simulink model "ACC_speed_change_curve_cs"  (R2016a)
settings: Solver=ode5  SolverMode=SingleTasking  StartTime=0.0  StopTime=inf  FixedStep=1/1000  RelTol=1e-3
PreLoadFcn:
  | mbxruntime.callbacks.PreLoadFcn(bdroot);
  | check_NUTS_defined;
  | 
  | assignin('base',['model_closed_' bdroot],false);addpath('../includes_ACC');
PostLoadFcn:
  | mbxruntime.callbacks.PostLoadFcn(bdroot);
InitFcn:
  | mbxruntime.callbacks.InitFcn(bdroot);
StartFcn:
  | mbxruntime.callbacks.StartFcn(bdroot);
StopFcn:
  | mbxruntime.callbacks.StopFcn(bdroot);
model workspace (MAT data in the model file):
  mbox_table : struct (value not decoded)
  model_closed = 0
  sim_status = 0
undefined symbols (not defined in the file or in its folder): DiscIntNeverNeededParam
undefined symbols (not defined in the file): SteeringColumn, SteeringWheel, WheelL0, WheelL1, WheelR0, WheelR1
libraries: simulink_extras x49, simulink x29, PreScanSimulinkLibrary x24, PreScanUsefulBlocks x2, Solver_SF x1, simulink_need_slupdate x1
(part 16 of 17)

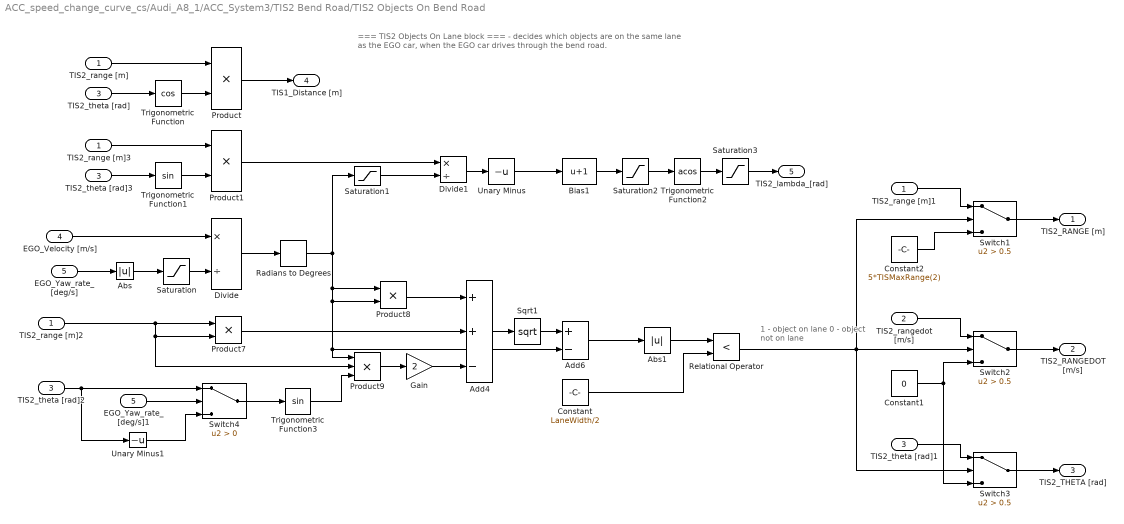
== system ACC_speed_change_curve_cs/Audi_A8_1/ACC_System3/TIS2 Bend Road/TIS2 Objects On Bend Road ==
  note: === TIS2 Objects On Lane block ===
      |
      |  - decides which objects are on the same lane as the EGO car,
      |     when the EGO car drives through the bend road.
  note: 1  - object      on lane
      | 0 - object not on lane
  TIS2_range [m] : Inport
  TIS2_rangedot [m/s] : Inport  Port=2
  TIS2_theta [rad] : Inport  Port=3
  EGO_Velocity [m/s] : Inport  Port=4
  EGO_Yaw_rate_[deg/s] : Inport  Port=5
  Abs : Abs
  Abs1 : Abs
  Add4 : Sum  Inputs=++-
  Add6 : Sum  Inputs=+-
  Bias1 : Bias  Bias=1
  Constant : Constant  Value=LaneWidth/2
  Constant1 : Constant  Value=0
  Constant2 : Constant  Value=5*TISMaxRange(2)
  Divide : Product  Inputs=*/
  Divide1 : Product  Inputs=*/
  EGO_Yaw_rate_[deg/s]1 : InportShadow  Port=5
  Gain : Gain  Gain=2
  Product{,1,7..8} (4 alike) : Product  RndMeth=Zero
  Product9 : Product  Inputs=3  RndMeth=Zero
  Radians to Degrees : simulink_extras/Transformations/Radians to Degrees
  Relational Operator : RelationalOperator  Operator=<  OutDataTypeStr=boolean
  Saturation : Saturate  UpperLimit=inf  LowerLimit=1e-6
  Saturation1 : Saturate  UpperLimit=inf  LowerLimit=1e-6
  Saturation2 : Saturate  UpperLimit=1  LowerLimit=-1
  Saturation3 : Saturate  UpperLimit=pi  LowerLimit=0
  Sqrt1 : Math  Operator=sqrt  SaturateOnIntegerOverflow=on
  Switch1 : Switch  Criteria=u2 > Threshold  Threshold=0.5
  Switch2 : Switch  Criteria=u2 > Threshold  Threshold=0.5
  Switch3 : Switch  Criteria=u2 > Threshold  Threshold=0.5
  Switch4 : Switch  Criteria=u2 > Threshold
  TIS2_range [m]1 : InportShadow
  TIS2_range [m]2 : InportShadow
  TIS2_range [m]3 : InportShadow
  TIS2_theta [rad]1 : InportShadow  Port=3
  TIS2_theta [rad]2 : InportShadow  Port=3
  TIS2_theta [rad]3 : InportShadow  Port=3
  Trigonometric Function : Trigonometry  Operator=cos
  Trigonometric Function1 : Trigonometry
  Trigonometric Function2 : Trigonometry  Operator=acos
  Trigonometric Function3 : Trigonometry
  Unary Minus : UnaryMinus
  Unary Minus1 : UnaryMinus
  TIS2_RANGE [m] : Outport
  TIS2_RANGEDOT [m/s] : Outport  Port=2
  TIS2_THETA [rad] : Outport  Port=3
  TIS1_Distance [m] : Outport  Port=4
  TIS2_lambda_[rad] : Outport  Port=5
  wires:
  Abs/1 -> Saturation/1
  Saturation3/1 -> TIS2_lambda_[rad]/1
  Saturation2/1 -> Trigonometric Function2/1
  Saturation1/1 -> Divide1/2
  Saturation/1 -> Divide/2
  Constant/1 -> Relational Operator/2
  Abs1/1 -> Relational Operator/1
  Product1/1 -> Divide1/1
  TIS2_theta [rad]3/1 -> Trigonometric Function1/1
  TIS2_range [m]3/1 -> Product1/1
  TIS2_range [m]2/1 -> Product9/2, Product7/2, Product7/1
  Unary Minus1/1 -> Switch4/3
  TIS2_theta [rad]2/1 -> Unary Minus1/1, Switch4/1
  Switch4/1 -> Trigonometric Function3/1
  EGO_Yaw_rate_[deg/s]1/1 -> Switch4/2
  Add6/1 -> Abs1/1
  Sqrt1/1 -> Add6/1
  Add4/1 -> Sqrt1/1
  Trigonometric Function3/1 -> Product9/3
  Product9/1 -> Gain/1
  Gain/1 -> Add4/3
  Product7/1 -> Add4/2
  Product8/1 -> Add4/1
  Product/1 -> TIS1_Distance [m]/1
  Trigonometric Function2/1 -> Saturation3/1
  Unary Minus/1 -> Bias1/1
  Divide1/1 -> Unary Minus/1
  Bias1/1 -> Saturation2/1
  Switch3/1 -> TIS2_THETA [rad]/1
  Switch2/1 -> TIS2_RANGEDOT [m/s]/1
  Switch1/1 -> TIS2_RANGE [m]/1
  Constant2/1 -> Switch1/3
  Constant1/1 -> Switch3/3, Switch2/3
  TIS2_theta [rad]1/1 -> Switch3/1
  TIS2_range [m]1/1 -> Switch1/1
  TIS2_rangedot [m/s]/1 -> Switch2/1
  Relational Operator/1 -> Switch3/2, Switch2/2, Switch1/2
  Radians to Degrees/1 -> Saturation1/1, Add6/2, Product9/1, Product8/2, Product8/1
  Divide/1 -> Radians to Degrees/1
  EGO_Yaw_rate_[deg/s]/1 -> Abs/1
  EGO_Velocity [m/s]/1 -> Divide/1
  Trigonometric Function1/1 -> Product1/2
  Trigonometric Function/1 -> Product/2
  TIS2_theta [rad]/1 -> Trigonometric Function/1
  TIS2_range [m]/1 -> Product/1

== system ACC_speed_change_curve_cs/Audi_A8_1/ACC_System3/TIS2 Bend Road/TIS2 Sorting Fun ==
  note: === TIS1 Sorting Fun block ===
      |
      |  - transforms information from the first sensor
      |    to the more appropriate form.
  TIS2range [m] : Inport
  TIS2rangedot [m/s] : Inport  Port=2
  TIS2theta [deg] : Inport  Port=3
  Degrees to Radians : simulink_extras/Transformations/Degrees to Radians
  Switch : Switch  Criteria=u2 ~= 0
  Unary Minus : UnaryMinus
  Unary Minus1 : UnaryMinus
  range max : Constant  Value=5*TISMaxRange(2)
  TIS2_RANGE [m] : Outport
  TIS2_RANGEDOT [m/s] : Outport  Port=2
  TIS2_THETA [rad] : Outport  Port=3
  wires:
  Unary Minus1/1 -> TIS2_RANGEDOT [m/s]/1
  TIS2theta [deg]/1 -> Unary Minus/1
  TIS2range [m]/1 -> Switch/1, Switch/2
  Degrees to Radians/1 -> TIS2_THETA [rad]/1
  range max/1 -> Switch/3
  TIS2rangedot [m/s]/1 -> Unary Minus1/1
  Switch/1 -> TIS2_RANGE [m]/1
  Unary Minus/1 -> Degrees to Radians/1

== system ACC_speed_change_curve_cs/Audi_A8_1/ACC_System3/TIS2 Straight Road/Hold ==
  HWTflagIN : Inport
  lead_vel_in : Inport  Port=2
  HWTflagIN1 : InportShadow
  If : If  IfExpression=u1 < 0.1  SampleTime=Tsensor
  If Action Subsystem : Subsystem  TreatAsAtomicUnit=on
  If Action Subsystem1 : Subsystem  TreatAsAtomicUnit=on
  Merge : Merge
  HWT_flag : Outport
  wires:
  HWTflagIN1/1 -> If Action Subsystem/1(In1)
  HWTflagIN/1 -> If Action Subsystem1/1(In1)
  Merge/1 -> HWT_flag/1
  If Action Subsystem1/1(Out1) -> Merge/2
  If Action Subsystem/1(Out1) -> Merge/1
  If/2 -> If Action Subsystem1/Action
  If/1 -> If Action Subsystem/Action
  lead_vel_in/1 -> If/1

== system ACC_speed_change_curve_cs/Audi_A8_1/ACC_System3/TIS2 Straight Road/TIS2 Closest Object ==
  note: === TIS2 Closest Object block ===
      |
      |  - passing through data about potentially the most dangerous object driving on the straight road.
  TIS2_rangedot [m/s] : Inport
  TIS2_distance [m] : Inport  Port=2
  index : Inport  Port=3
  Selector1 : Selector  InputPortWidth=TISdet(2)  IndexOptions=Index vector (port)  Indices=[1 3]  OutputSizes=1
  Selector2 : Selector  InputPortWidth=TISdet(2)  IndexOptions=Index vector (port)  Indices=[1 3]  OutputSizes=1
  rangedot [m/s] : Outport
  distance [m/s] : Outport  Port=2
  wires:
  index/1 -> Selector2/2, Selector1/2
  TIS2_rangedot [m/s]/1 -> Selector1/1
  Selector1/1 -> rangedot [m/s]/1
  TIS2_distance [m]/1 -> Selector2/1
  Selector2/1 -> distance [m/s]/1

== system ACC_speed_change_curve_cs/Audi_A8_1/ACC_System3/TIS2 Straight Road/TIS2 HWT Computing ==
  note: === TIS1 HWT Computing block===
      |
      |  - computes HeadWay Time (HWT) as it is defined in ISO norms.
  Distance [m] : Inport
  HWT demanded : Inport  Port=2
  Velocity [m/s] : Inport  Port=3
  If : If
  If Action Subsystem : Subsystem  TreatAsAtomicUnit=on
  If Action Subsystem1 : Subsystem  TreatAsAtomicUnit=on
  Merge : Merge
  HWT [s] : Outport
  wires:
  HWT demanded/1 -> If Action Subsystem1/1(HWT demanded [s])
  Distance [m]/1 -> If Action Subsystem/1(Distance [m])
  Merge/1 -> HWT [s]/1
  If Action Subsystem1/1(Out1) -> Merge/2
  If Action Subsystem/1(HWT [s]) -> Merge/1
  If/2 -> If Action Subsystem1/Action
  If/1 -> If Action Subsystem/Action
  Velocity [m/s]/1 -> If Action Subsystem/2(Velocity [m/s]), If/1

== system ACC_speed_change_curve_cs/Audi_A8_1/ACC_System3/TIS2 Straight Road/TIS2 HWT Computing2 ==
  note: === TIS1 HWT Computing block===
      |
      |  - computes HeadWay Time (HWT) as it is defined in ISO norms.
  Distance [m] : Inport
  Velocity [m/s] : Inport  Port=2
  If : If
  If Action Subsystem : Subsystem  TreatAsAtomicUnit=on
  If Action Subsystem1 : Subsystem  TreatAsAtomicUnit=on
  Merge : Merge
  HWT [s] : Outport
  wires:
  Distance [m]/1 -> If Action Subsystem/1(Distance [m])
  Merge/1 -> HWT [s]/1
  If Action Subsystem1/1(Out1) -> Merge/2
  If Action Subsystem/1(HWT [s]) -> Merge/1
  If/2 -> If Action Subsystem1/Action
  If/1 -> If Action Subsystem/Action
  Velocity [m/s]/1 -> If Action Subsystem/2(Velocity [m/s]), If/1

== system ACC_speed_change_curve_cs/Audi_A8_1/ACC_System3/TIS2 Straight Road/TIS2 HWT Flag ==
  note: === TIS2 HWT Flag block ===
      |
      |  - outputs the HeadWay Time (HWT) flag,
      |  - holds a high level if the criteria were met,
      |  - sets HWT flag to low level if leading car
      |    went outside the scope of the sensors.
  Distance closest [m] : Inport
  HWT_dem [s] : Inport  Port=2
  HWT [s] : Inport  Port=3
  Standstill distance : Inport  Port=4
  Abs : Abs
  Compare To Constant1 : simulink/Logic and Bit Operations/Compare To Constant  relop===  const=5*TISMaxRange(2)  OutDataTypeStr=uint8
  Constant : Constant
  Constant1 : Constant  Value=0
  Data Type Conversion : DataTypeConversion
  Data Type Conversion1 : DataTypeConversion
  Discrete-Time Integrator : DiscreteIntegrator  ExternalReset=level  SampleTime=Tsensor  ICPrevOutput=DiscIntNeverNeededParam  ICPrevScaledInput=DiscIntNeverNeededParam
  Distance closest [m]1 : InportShadow
  Gain : Gain  Gain=2
  Gain1 : Gain
  Gain2 : Gain  Gain=1e6  OutDataTypeStr=double
  Gain3 : Gain  Gain=1e6  OutDataTypeStr=double
  Gain4 : Gain  Gain=1.25
  Gain6 : Gain  Gain=100
  Gain7 : Gain  Gain=1.25
  Gain8 : Gain  Gain=0.01
  HWT [s]1 : InportShadow  Port=3
  HWT [s]3 : InportShadow  Port=3
  HWT_dem [s]1 : InportShadow  Port=2
  HWT_dem [s]2 : InportShadow  Port=2
  Logical Operator : Logic  AllPortsSameDT=off  OutDataTypeStr=boolean
  Logical Operator1 : Logic  AllPortsSameDT=off  OutDataTypeStr=boolean
  Logical Operator2 : Logic  Operator=OR  Inputs=3  AllPortsSameDT=off  OutDataTypeStr=boolean
  Logical Operator3 : Logic  AllPortsSameDT=off  OutDataTypeStr=boolean
  MinMax : MinMax
  MinMax2 : MinMax
  Relational Operator : RelationalOperator  Operator=<=  OutDataTypeStr=boolean
  Relational Operator1 : RelationalOperator  OutDataTypeStr=boolean
  Relational Operator2 : RelationalOperator  Operator=>  OutDataTypeStr=boolean
  Relational Operator4 : RelationalOperator  Operator=>  OutDataTypeStr=boolean
  Rounding Function : Rounding
  Sum of Elements : Sum  Inputs=+
  Switch : Switch  Criteria=u2 > Threshold
  HWT_flag : Outport
  wires:
  Data Type Conversion1/1 -> Gain3/1
  Data Type Conversion/1 -> Gain2/1
  Relational Operator4/1 -> Logical Operator2/3
  Gain7/1 -> Relational Operator4/2
  Gain8/1 -> Relational Operator4/1
  MinMax2/1 -> Gain6/1
  Rounding Function/1 -> Gain8/1
  Gain6/1 -> Rounding Function/1
  HWT [s]3/1 -> MinMax2/1
  HWT_dem [s]2/1 -> Gain7/1
  Gain4/1 -> Relational Operator/2
  Switch/1 -> HWT_flag/1
  Constant1/1 -> Switch/3
  Constant/1 -> Switch/1
  Abs/1 -> Switch/2
  Discrete-Time Integrator/1 -> Abs/1
  Gain3/1 -> Discrete-Time Integrator/1
  Gain2/1 -> Discrete-Time Integrator/2
  Logical Operator3/1 -> Logical Operator2/2
  MinMax/1 -> Logical Operator3/1
  Relational Operator2/1 -> Logical Operator3/2
  Standstill distance/1 -> Relational Operator2/2
  Distance closest [m]1/1 -> Relational Operator2/1
  HWT_dem [s]1/1 -> Gain/1
  Logical Operator2/1 -> Data Type Conversion/1
  Gain1/1 -> MinMax/1
  Relational Operator1/1 -> Gain1/1
  Gain/1 -> Relational Operator1/2
  HWT [s]1/1 -> Relational Operator1/1
  Compare To Constant1/1 -> Logical Operator1/1, Logical Operator1/2
  HWT [s]/1 -> Relational Operator/1
  HWT_dem [s]/1 -> Gain4/1
  Relational Operator/1 -> Sum of Elements/1
  Sum of Elements/1 -> Logical Operator/1, Logical Operator/2
  Logical Operator/1 -> Data Type Conversion1/1
  Distance closest [m]/1 -> Compare To Constant1/1
  Logical Operator1/1 -> Logical Operator2/1

== system ACC_speed_change_curve_cs/Audi_A8_1/ACC_System3/TIS2 Straight Road/TIS2 Lead Car Longitudinal Velocity ==
  note: === TIS2 Lead Car Longitudinal Velocity block ===
      |
      |  - computes the leading car absolute velocity and safe distance between the EGO and leading car.
  HWT_dem (s) : Inport
  TIS2 Rangedot [m/s] : Inport  Port=2
  EGO Velocity [m/s] : Inport  Port=3
  Standstill [m] : Inport  Port=4
  Abs : Abs
  Add : Sum  Inputs=+-
  Constant : Constant  Value=0
  Divide : Product  Inputs=*/
  HWT_dem (s)1 : InportShadow
  Product : Product  RndMeth=Zero
  Relational Operator : RelationalOperator  Operator=<=  OutDataTypeStr=boolean
  Switch : Switch  Criteria=u2 > Threshold
  Switch1 : Switch  Criteria=u2 ~= 0
  TIS2 Rangedot [m/s]1 : InportShadow  Port=2
  Safe distance [m] : Outport
  Lead velocity [m/s] : Outport  Port=2
  wires:
  Abs/1 -> Switch1/1, Relational Operator/1, Product/1
  TIS2 Rangedot [m/s]1/1 -> Switch1/2
  Switch1/1 -> Lead velocity [m/s]/1
  Constant/1 -> Switch1/3
  EGO Velocity [m/s]/1 -> Add/1
  TIS2 Rangedot [m/s]/1 -> Add/2
  Add/1 -> Abs/1
  HWT_dem (s)/1 -> Product/2
  Product/1 -> Switch/3
  Switch/1 -> Safe distance [m]/1
  Standstill [m]/1 -> Divide/1, Switch/1
  HWT_dem (s)1/1 -> Divide/2
  Divide/1 -> Relational Operator/2
  Relational Operator/1 -> Switch/2

== system ACC_speed_change_curve_cs/Audi_A8_1/ACC_System3/TIS2 Straight Road/TIS2 Objects On Lane ==
  note: === TIS2 Objects On Lane block ===
      |
      |  - decides which objects are on the same lane as the EGO car,
      |    when the EGO car drives straight.
  TIS2_range [m] : Inport
  TIS2_rangedot [m/s] : Inport  Port=2
  TIS2_theta [rad] : Inport  Port=3
  Abs : Abs
  Compare To Constant : simulink/Logic and Bit Operations/Compare To Constant  relop=<  const=LaneWidth/2  OutDataTypeStr=boolean
  Constant : Constant  Value=0
  Product : Product  RndMeth=Zero
  Product1 : Product  RndMeth=Zero
  Switch1 : Switch  Criteria=u2 > Threshold  Threshold=0.5
  Switch3 : Switch  Criteria=u2 > Threshold  Threshold=0.5
  TIS2 range max (higher value) : Constant  Value=5*TISMaxRange(2)
  Trigonometric Function : Trigonometry
  Trigonometric Function1 : Trigonometry  Operator=cos
  TIS2_RANGEDOT [m/s] : Outport
  TIS2_Distance [m] : Outport  Port=2
  wires:
  TIS2_theta [rad]/1 -> Abs/1, Trigonometric Function1/1
  Trigonometric Function/1 -> Product/2
  Product/1 -> Compare To Constant/1
  TIS2_range [m]/1 -> Product1/1, Product/1
  TIS2_rangedot [m/s]/1 -> Switch1/1
  Switch1/1 -> TIS2_RANGEDOT [m/s]/1
  Switch3/1 -> TIS2_Distance [m]/1
  Abs/1 -> Trigonometric Function/1
  Trigonometric Function1/1 -> Product1/2
  Product1/1 -> Switch3/1
  TIS2 range max (higher value)/1 -> Switch3/3
  Constant/1 -> Switch1/3
  Compare To Constant/1 -> Switch3/2, Switch1/2

== system ACC_speed_change_curve_cs/Audi_A8_1/ACC_System3/TIS2 Straight Road/TIS2 Sorting Fun ==
  note: === TIS2 Sorting Fun block ===
      |
      |  - transforms information from the second sensor
      |    to the more appropriate form.
  TIS2range [m] : Inport
  TIS2rangedot [m/s] : Inport  Port=2
  TIS2theta [deg] : Inport  Port=3
  Degrees to Radians : simulink_extras/Transformations/Degrees to Radians
  Switch : Switch  Criteria=u2 ~= 0
  Unary Minus : UnaryMinus
  Unary Minus1 : UnaryMinus
  range max (higher value which will not generate high level of HWT flag) : Constant  Value=5*TISMaxRange(2)
  TIS2_RANGE [m] : Outport
  TIS2_RANGEDOT [m/s] : Outport  Port=2
  TIS2_THETA [rad] : Outport  Port=3
  wires:
  Unary Minus/1 -> Degrees to Radians/1
  Switch/1 -> TIS2_RANGE [m]/1
  TIS2rangedot [m/s]/1 -> Unary Minus1/1
  range max (higher value which will not generate high level of HWT flag)/1 -> Switch/3
  Degrees to Radians/1 -> TIS2_THETA [rad]/1
  TIS2range [m]/1 -> Switch/1, Switch/2
  TIS2theta [deg]/1 -> Unary Minus/1
  Unary Minus1/1 -> TIS2_RANGEDOT [m/s]/1

== system ACC_speed_change_curve_cs/Audi_A8_1/CarSim2PreScan/Transformation_WheelGlobal2WheelLocal/Subsystem ==
  Wheels_Pos_Global_xyz_[m] : Inport
  In2 : Inport  Port=2
  In3 : Inport  Port=3
  In4 : Inport  Port=4
  Demux1 : Demux  Outputs=[3 3 3 3]
  Dot Product{1..12} (12 alike) : DotProduct  InputSameDT=on  OutDataTypeStr=Inherit: Inherit via internal rule
  Mux{1..4} (4 alike) : Mux  Inputs=3
  FL_xyz : Outport
  FR_xyz : Outport  Port=2
  RL_xyz : Outport  Port=3
  RR_xyz : Outport  Port=4
  wires:
  [ThirdRow] -> Dot Product12/2
  [ThirdRow] -> Dot Product9/2
  [ThirdRow] -> Dot Product6/2
  [SecondRow] -> Dot Product11/2
  [SecondRow] -> Dot Product8/2
  [SecondRow] -> Dot Product5/2
  In2/1 -> [FirstRow], Dot Product1/2
  [FirstRow] -> Dot Product10/2
  [FirstRow] -> Dot Product7/2
  [FirstRow] -> Dot Product4/2
  Demux1/4 -> Dot Product12/1, Dot Product10/1, Dot Product11/1
  Demux1/3 -> Dot Product9/1, Dot Product7/1, Dot Product8/1
  Demux1/2 -> Dot Product6/1, Dot Product5/1, Dot Product4/1
  Demux1/1 -> Dot Product3/1, Dot Product2/1, Dot Product1/1
  Mux4/1 -> RR_xyz/1
  Dot Product11/1 -> Mux4/2
  Dot Product12/1 -> Mux4/3
  Dot Product10/1 -> Mux4/1
  Mux3/1 -> RL_xyz/1
  Dot Product8/1 -> Mux3/2
  Dot Product9/1 -> Mux3/3
  Dot Product7/1 -> Mux3/1
  Mux1/1 -> FR_xyz/1
  Dot Product5/1 -> Mux1/2
  Dot Product6/1 -> Mux1/3
  Dot Product4/1 -> Mux1/1
  Mux2/1 -> FL_xyz/1
  Dot Product2/1 -> Mux2/2
  Dot Product3/1 -> Mux2/3
  Dot Product1/1 -> Mux2/1
  Wheels_Pos_Global_xyz_[m]/1 -> Demux1/1
  In4/1 -> [ThirdRow], Dot Product3/2
  In3/1 -> [SecondRow], Dot Product2/2

== system ACC_speed_change_curve_cs/Audi_A8_1/PathFollower_1/CTRL REFERENCES/Calculate Preview Point (pvp) by extrapolating current Vehicle Position (p0) with Preview Distance and Vehicle Orientation ==
  Preview Distance : Inport
  x,y,Y Demux [m,m,rad] : Inport  Port=2
  Demux : Demux  Outputs=3
  Fcn : Fcn  Expr=u(2)*cos(u(1))
  Fcn1 : Fcn  Expr=u(2)*sin(u(1))
  Mux : Mux  Inputs=2
  Sum : Sum  Inputs=|++
  Sum1 : Sum  Inputs=|++
  x_glob_PVD : Outport
  y_glob_PVD : Outport  Port=2
  Y [rad] : Outport  Port=3
  wires:
  Demux/3 -> Mux/1, Y [rad]/1
  Demux/1 -> Sum/1
  Demux/2 -> Sum1/1
  Preview Distance/1 -> Mux/2
  Mux/1 -> Fcn/1, Fcn1/1
  Fcn/1 -> Sum/2
  Fcn1/1 -> Sum1/2
  Sum/1 -> x_glob_PVD/1
  Sum1/1 -> y_glob_PVD/1
  x,y,Y Demux [m,m,rad]/1 -> Demux/1

== system ACC_speed_change_curve_cs/Audi_A8_1/PathFollower_1/CTRL REFERENCES/Find Reference Point (pref) on Trajectory closest to PVP Point (pvp) ==
  In1 : Inport
  In2 : Inport  Port=2
  In3 : Inport  Port=3
  In4 : Inport  Port=4
  eml_find_closest_trajectory_points : MATLAB Function  TreatAsAtomicUnit=on
  Out1 : Outport
  Out2 : Outport  Port=2
  Out3 : Outport  Port=3
  wires:
  eml_find_closest_trajectory_points/3(Actor_traj_angle) -> Out3/1
  eml_find_closest_trajectory_points/2(Actor_traj_distance) -> Out2/1
  eml_find_closest_trajectory_points/1(pref) -> Out1/1
  In1/1 -> eml_find_closest_trajectory_points/1(pvp)
  In2/1 -> eml_find_closest_trajectory_points/2(TrajOffset_x_y_Y)
  In3/1 -> eml_find_closest_trajectory_points/3(ActorOffset_Left_Right)
  In4/1 -> eml_find_closest_trajectory_points/4(p0)

== system ACC_speed_change_curve_cs/Audi_A8_1/PathFollower_1/DELTA CTRL/Calculate preview angle ==
  In1 : Inport
  In2 : Inport  Port=2
  In3 : Inport  Port=3
  eml_preview_angle_and_distance : MATLAB Function  TreatAsAtomicUnit=on
  Out1 : Outport
  wires:
  In3/1 -> eml_preview_angle_and_distance/3(p0)
  In2/1 -> eml_preview_angle_and_distance/2(pref)
  In1/1 -> eml_preview_angle_and_distance/1(pvp)
  eml_preview_angle_and_distance/1(alpha) -> Out1/1

== system ACC_speed_change_curve_cs/Audi_A8_1/PathFollower_1/DELTA CTRL/Error check ==
  Add3 : Sum  Inputs=-+
  Demux : Demux  Outputs=2
  Selector1 : Selector  InputPortWidth=3  IndexOptions=Index vector (dialog)  Indices=[1 2]  OutputSizes=1
  p0_x error : Scope
  p0_y error : Scope
  wires:
  Demux/2 -> p0_y error/1
  Add3/1 -> Demux/1
  Demux/1 -> p0_x error/1
  [pref0] -> Add3/2
  [p0] -> Selector1/1
  Selector1/1 -> Add3/1

== system ACC_speed_change_curve_cs/Audi_A8_1/PathFollower_1/THROTTLE CTRL/If Desired Velocity = 0 ==
  In1 : Inport
  Action Port : ActionPort  InitializeStates=reset  PropagateVarSize=During execution  ActionType=then
  constant : Constant  Value=0
  constant1 : Constant  Value=150
  throttle [%] : Outport  InitialOutput=[0]
  brake pressure [bar] : Outport  Port=2  InitialOutput=[150]
  Auto_GearShift : Outport  Port=3
  wires:
  constant1/1 -> brake pressure [bar]/1
  constant/1 -> throttle [%]/1
  In1/1 -> Auto_GearShift/1

== system ACC_speed_change_curve_cs/Audi_A8_1/PathFollower_1/THROTTLE CTRL/If Desired Velocity ~= 0 ==
  note: CONSTANT VELOCITY CONTROL
  note: No brake/throttle actions
      | in case of small ctrl error,
      |  in order to prevent nervous
      | ctrl behaviour
  In1 : Inport
  Desired Velocity [m/s] : Inport  Port=2
  Action Port : ActionPort  InitializeStates=reset  PropagateVarSize=During execution  ActionType=else
  Dead Zone : DeadZone  LowerValue=-10  UpperValue=1  SaturateOnIntegerOverflow=on
  Gain11 : Gain  Gain=10
  Gain6 : Gain  Gain=-1
  Limiter_brake : Saturate  UpperLimit=150  LowerLimit=0
  Limiter_throttle : Saturate  UpperLimit=100  LowerLimit=0
  PID Controller : simulink_need_slupdate/PID Controller  P=20  I=0.3  D=3.065
  throttle [%] : Outport
  brake pressure [bar] : Outport  Port=2
  Auto_GearShift : Outport  Port=3
  wires:
  Limiter_throttle/1 -> throttle [%]/1  "throttle"
  Limiter_brake/1 -> brake pressure [bar]/1
  Gain6/1 -> Limiter_brake/1
  Gain11/1 -> Gain6/1
  Dead Zone/1 -> Limiter_throttle/1, Gain11/1
  Desired Velocity [m/s]/1 -> PID Controller/1
  PID Controller/1 -> Dead Zone/1
  In1/1 -> Auto_GearShift/1

== system ACC_speed_change_curve_cs/Audi_A8_1/SELF_Demux/compas converter/cart2compas ==
  Angle [deg] : Inport
  Constant : Constant  Value=90
  Constant1 : Constant  Value=360
  Gain : Gain  Gain=1/360
  Gain1 : Gain  Gain=360
  Gain2 : Gain  Gain=-1
  Rounding Function : Rounding
  Sum : Sum  Inputs=|-+
  Sum1 : Sum  Inputs=-+|
  Sum2 : Sum  Inputs=++|
  heading [deg] : Outport
  wires:
  Gain/1 -> Rounding Function/1
  Rounding Function/1 -> Gain1/1
  Gain1/1 -> Sum/1
  Angle [deg]/1 -> Sum1/2
  Sum/1 -> Gain2/1
  Sum1/1 -> Gain/1, Sum/2
  Constant/1 -> Sum1/1
  Gain2/1 -> Sum2/2
  Constant1/1 -> Sum2/1
  Sum2/1 -> heading [deg]/1

== system ACC_speed_change_curve_cs/Audi_A8_1/Trajectories/Traj2State1/Traj2State2 ==
  traj : Inport
  MuxState : Subsystem
  Traj2MuxState_Ext : Subsystem
  state : Outport
  wires:
  Traj2MuxState_Ext/9(Y [rad]) -> MuxState/9(Y [rad])
  Traj2MuxState_Ext/8(P [rad]) -> MuxState/8(P [rad])
  Traj2MuxState_Ext/7(R [rad]) -> MuxState/7(R [rad])
  Traj2MuxState_Ext/6(dz [m/s]) -> MuxState/6(dz [m/s])
  Traj2MuxState_Ext/5(dy [m/s]) -> MuxState/5(dy [m/s])
  Traj2MuxState_Ext/4(dx [m/s]) -> MuxState/4(dx [m/s])
  Traj2MuxState_Ext/3(z [m]) -> MuxState/3(z [m])
  Traj2MuxState_Ext/2(y [m]) -> MuxState/2(y [m])
  Traj2MuxState_Ext/1(x [m]) -> MuxState/1(x [m])
  MuxState/1(state) -> state/1
  traj/1 -> Traj2MuxState_Ext/1(Traj)

== system ACC_speed_change_curve_cs/BMW_X5_1/SELF_Demux/compas converter/cart2compas ==
  Angle [deg] : Inport
  Constant : Constant  Value=90
  Constant1 : Constant  Value=360
  Gain : Gain  Gain=1/360
  Gain1 : Gain  Gain=360
  Gain2 : Gain  Gain=-1
  Rounding Function : Rounding
  Sum : Sum  Inputs=|-+
  Sum1 : Sum  Inputs=-+|
  Sum2 : Sum  Inputs=++|
  heading [deg] : Outport
  wires:
  Gain/1 -> Rounding Function/1
  Rounding Function/1 -> Gain1/1
  Gain1/1 -> Sum/1
  Angle [deg]/1 -> Sum1/2
  Sum/1 -> Gain2/1
  Sum1/1 -> Gain/1, Sum/2
  Constant/1 -> Sum1/1
  Gain2/1 -> Sum2/2
  Constant1/1 -> Sum2/1
  Sum2/1 -> heading [deg]/1

== system ACC_speed_change_curve_cs/BMW_X5_1/Trajectories/Traj2State1/Traj2State2 ==
  traj : Inport
  MuxState : Subsystem
  Traj2MuxState_Ext : Subsystem
  state : Outport
  wires:
  Traj2MuxState_Ext/9(Y [rad]) -> MuxState/9(Y [rad])
  Traj2MuxState_Ext/8(P [rad]) -> MuxState/8(P [rad])
  Traj2MuxState_Ext/7(R [rad]) -> MuxState/7(R [rad])
  Traj2MuxState_Ext/6(dz [m/s]) -> MuxState/6(dz [m/s])
  Traj2MuxState_Ext/5(dy [m/s]) -> MuxState/5(dy [m/s])
  Traj2MuxState_Ext/4(dx [m/s]) -> MuxState/4(dx [m/s])
  Traj2MuxState_Ext/3(z [m]) -> MuxState/3(z [m])
  Traj2MuxState_Ext/2(y [m]) -> MuxState/2(y [m])
  Traj2MuxState_Ext/1(x [m]) -> MuxState/1(x [m])
  MuxState/1(state) -> state/1
  traj/1 -> Traj2MuxState_Ext/1(Traj)

== system ACC_speed_change_curve_cs/Toyota_Previa_1/SELF_Demux/compas converter/cart2compas ==
  Angle [deg] : Inport
  Constant : Constant  Value=90
  Constant1 : Constant  Value=360
  Gain : Gain  Gain=1/360
  Gain1 : Gain  Gain=360
  Gain2 : Gain  Gain=-1
  Rounding Function : Rounding
  Sum : Sum  Inputs=|-+
  Sum1 : Sum  Inputs=-+|
  Sum2 : Sum  Inputs=++|
  heading [deg] : Outport
  wires:
  Gain/1 -> Rounding Function/1
  Rounding Function/1 -> Gain1/1
  Gain1/1 -> Sum/1
  Angle [deg]/1 -> Sum1/2
  Sum/1 -> Gain2/1
  Sum1/1 -> Gain/1, Sum/2
  Constant/1 -> Sum1/1
  Gain2/1 -> Sum2/2
  Constant1/1 -> Sum2/1
  Sum2/1 -> heading [deg]/1

== system ACC_speed_change_curve_cs/Toyota_Previa_1/Trajectories/Traj2State1/Traj2State2 ==
  traj : Inport
  MuxState : Subsystem
  Traj2MuxState_Ext : Subsystem
  state : Outport
  wires:
  Traj2MuxState_Ext/9(Y [rad]) -> MuxState/9(Y [rad])
  Traj2MuxState_Ext/8(P [rad]) -> MuxState/8(P [rad])
  Traj2MuxState_Ext/7(R [rad]) -> MuxState/7(R [rad])
  Traj2MuxState_Ext/6(dz [m/s]) -> MuxState/6(dz [m/s])
  Traj2MuxState_Ext/5(dy [m/s]) -> MuxState/5(dy [m/s])
  Traj2MuxState_Ext/4(dx [m/s]) -> MuxState/4(dx [m/s])
  Traj2MuxState_Ext/3(z [m]) -> MuxState/3(z [m])
  Traj2MuxState_Ext/2(y [m]) -> MuxState/2(y [m])
  Traj2MuxState_Ext/1(x [m]) -> MuxState/1(x [m])
  MuxState/1(state) -> state/1
  traj/1 -> Traj2MuxState_Ext/1(Traj)

== system ACC_speed_change_curve_cs/Toyota_Yaris_1/SELF_Demux/compas converter/cart2compas ==
  Angle [deg] : Inport
  Constant : Constant  Value=90
  Constant1 : Constant  Value=360
  Gain : Gain  Gain=1/360
  Gain1 : Gain  Gain=360
  Gain2 : Gain  Gain=-1
  Rounding Function : Rounding
  Sum : Sum  Inputs=|-+
  Sum1 : Sum  Inputs=-+|
  Sum2 : Sum  Inputs=++|
  heading [deg] : Outport
  wires:
  Gain/1 -> Rounding Function/1
  Rounding Function/1 -> Gain1/1
  Gain1/1 -> Sum/1
  Angle [deg]/1 -> Sum1/2
  Sum/1 -> Gain2/1
  Sum1/1 -> Gain/1, Sum/2
  Constant/1 -> Sum1/1
  Gain2/1 -> Sum2/2
  Constant1/1 -> Sum2/1
  Sum2/1 -> heading [deg]/1

== system ACC_speed_change_curve_cs/Toyota_Yaris_1/Trajectories/Traj2State1/Traj2State2 ==
  traj : Inport
  MuxState : Subsystem
  Traj2MuxState_Ext : Subsystem
  state : Outport
  wires:
  Traj2MuxState_Ext/9(Y [rad]) -> MuxState/9(Y [rad])
  Traj2MuxState_Ext/8(P [rad]) -> MuxState/8(P [rad])
  Traj2MuxState_Ext/7(R [rad]) -> MuxState/7(R [rad])
  Traj2MuxState_Ext/6(dz [m/s]) -> MuxState/6(dz [m/s])
  Traj2MuxState_Ext/5(dy [m/s]) -> MuxState/5(dy [m/s])
  Traj2MuxState_Ext/4(dx [m/s]) -> MuxState/4(dx [m/s])
  Traj2MuxState_Ext/3(z [m]) -> MuxState/3(z [m])
  Traj2MuxState_Ext/2(y [m]) -> MuxState/2(y [m])
  Traj2MuxState_Ext/1(x [m]) -> MuxState/1(x [m])
  MuxState/1(state) -> state/1
  traj/1 -> Traj2MuxState_Ext/1(Traj)

== system ACC_speed_change_curve_cs/Audi_A8_1/ACC_System/TIS1 Bend Road/Hold/If Action Subsystem ==
  In1 : Inport
  Action Port : ActionPort  InitializeStates=reset  PropagateVarSize=During execution  ActionType=then
  Constant : Constant
  Constant1 : Constant  Value=0
  Discrete-Time Integrator : DiscreteIntegrator  gainval=100  InitialConditionSource=external  InitialConditionSetting=State (most efficient)  SampleTime=Tsensor  LimitOutput=on  UpperSaturationLimit=1  LowerSaturationLimit=0  ICPrevOutput=DiscIntNeverNeededParam  ICPrevScaledInput=DiscIntNeverNeededParam
  Gain3 : Gain  Gain=1e6  OutDataTypeStr=double
  Switch : Switch  Criteria=u2 > Threshold
  Out1 : Outport
  wires:
  Gain3/1 -> Discrete-Time Integrator/1
  In1/1 -> Gain3/1, Switch/2
  Discrete-Time Integrator/1 -> Out1/1
  Switch/1 -> Discrete-Time Integrator/2
  Constant/1 -> Switch/1
  Constant1/1 -> Switch/3

== system ACC_speed_change_curve_cs/Audi_A8_1/ACC_System/TIS1 Bend Road/Hold/If Action Subsystem1 ==
  In1 : Inport
  Action Port : ActionPort  PropagateVarSize=During execution  ActionType=else
  Out1 : Outport
  wires:
  In1/1 -> Out1/1

== system ACC_speed_change_curve_cs/Audi_A8_1/ACC_System/TIS1 Bend Road/TIS1 HWT Computing/If Action Subsystem ==
  Distance [m] : Inport
  Velocity [m/s] : Inport  Port=2
  Action Port : ActionPort  PropagateVarSize=During execution  ActionType=then
  Product : Product  Inputs=*/  RndMeth=Zero
  HWT [s] : Outport
  wires:
  Distance [m]/1 -> Product/1
  Velocity [m/s]/1 -> Product/2
  Product/1 -> HWT [s]/1

== system ACC_speed_change_curve_cs/Audi_A8_1/ACC_System/TIS1 Bend Road/TIS1 HWT Computing/If Action Subsystem1 ==
  Action Port : ActionPort  PropagateVarSize=During execution  ActionType=else
  Constant : Constant  Value=inf
  Out1 : Outport  InitialOutput=0
  wires:
  Constant/1 -> Out1/1

== system ACC_speed_change_curve_cs/Audi_A8_1/ACC_System/TIS1 Straight Road/Hold/If Action Subsystem ==
  In1 : Inport
  Action Port : ActionPort  InitializeStates=reset  PropagateVarSize=During execution  ActionType=then
  Constant : Constant
  Constant1 : Constant  Value=0
  Discrete-Time Integrator : DiscreteIntegrator  gainval=100  InitialConditionSource=external  InitialConditionSetting=State (most efficient)  SampleTime=Tsensor  LimitOutput=on  UpperSaturationLimit=1  LowerSaturationLimit=0  ICPrevOutput=DiscIntNeverNeededParam  ICPrevScaledInput=DiscIntNeverNeededParam
  Gain3 : Gain  Gain=1e6  OutDataTypeStr=double
  Switch : Switch  Criteria=u2 > Threshold
  Out1 : Outport
  wires:
  Gain3/1 -> Discrete-Time Integrator/1
  In1/1 -> Gain3/1, Switch/2
  Discrete-Time Integrator/1 -> Out1/1
  Switch/1 -> Discrete-Time Integrator/2
  Constant/1 -> Switch/1
  Constant1/1 -> Switch/3

== system ACC_speed_change_curve_cs/Audi_A8_1/ACC_System/TIS1 Straight Road/Hold/If Action Subsystem1 ==
  In1 : Inport
  Action Port : ActionPort  PropagateVarSize=During execution  ActionType=else
  Out1 : Outport
  wires:
  In1/1 -> Out1/1

== system ACC_speed_change_curve_cs/Audi_A8_1/ACC_System/TIS1 Straight Road/TIS1 HWT Computing/If Action Subsystem ==
  Distance [m] : Inport
  Velocity [m/s] : Inport  Port=2
  Action Port : ActionPort  PropagateVarSize=During execution  ActionType=then
  Product : Product  Inputs=*/  RndMeth=Zero
  HWT [s] : Outport
  wires:
  Distance [m]/1 -> Product/1
  Velocity [m/s]/1 -> Product/2
  Product/1 -> HWT [s]/1

== system ACC_speed_change_curve_cs/Audi_A8_1/ACC_System/TIS1 Straight Road/TIS1 HWT Computing/If Action Subsystem1 ==
  HWT demanded [s] : Inport
  Action Port : ActionPort  PropagateVarSize=During execution  ActionType=else
  Gain : Gain  Gain=2*ones(TISdet(1),1)
  Out1 : Outport
  wires:
  Gain/1 -> Out1/1
  HWT demanded [s]/1 -> Gain/1

== system ACC_speed_change_curve_cs/Audi_A8_1/ACC_System/TIS1 Straight Road/TIS1 HWT Computing1/If Action Subsystem ==
  Distance [m] : Inport
  Velocity [m/s] : Inport  Port=2
  Action Port : ActionPort  PropagateVarSize=During execution  ActionType=then
  Product : Product  Inputs=*/  RndMeth=Zero
  HWT [s] : Outport
  wires:
  Distance [m]/1 -> Product/1
  Velocity [m/s]/1 -> Product/2
  Product/1 -> HWT [s]/1

== system ACC_speed_change_curve_cs/Audi_A8_1/ACC_System/TIS1 Straight Road/TIS1 HWT Computing1/If Action Subsystem1 ==
  Action Port : ActionPort  PropagateVarSize=During execution  ActionType=else
  Constant : Constant  Value=inf
  Out1 : Outport  InitialOutput=0
  wires:
  Constant/1 -> Out1/1

== system ACC_speed_change_curve_cs/Audi_A8_1/ACC_System/TIS2 Bend Road/Hold/If Action Subsystem ==
  In1 : Inport
  Action Port : ActionPort  InitializeStates=reset  PropagateVarSize=During execution  ActionType=then
  Constant : Constant
  Constant1 : Constant  Value=0
  Discrete-Time Integrator : DiscreteIntegrator  gainval=100  InitialConditionSource=external  InitialConditionSetting=State (most efficient)  SampleTime=Tsensor  LimitOutput=on  UpperSaturationLimit=1  LowerSaturationLimit=0  ICPrevOutput=DiscIntNeverNeededParam  ICPrevScaledInput=DiscIntNeverNeededParam
  Gain3 : Gain  Gain=1e6  OutDataTypeStr=double
  Switch : Switch  Criteria=u2 > Threshold
  Out1 : Outport
  wires:
  Gain3/1 -> Discrete-Time Integrator/1
  In1/1 -> Gain3/1, Switch/2
  Discrete-Time Integrator/1 -> Out1/1
  Switch/1 -> Discrete-Time Integrator/2
  Constant/1 -> Switch/1
  Constant1/1 -> Switch/3

== system ACC_speed_change_curve_cs/Audi_A8_1/ACC_System/TIS2 Bend Road/Hold/If Action Subsystem1 ==
  In1 : Inport
  Action Port : ActionPort  PropagateVarSize=During execution  ActionType=else
  Out1 : Outport
  wires:
  In1/1 -> Out1/1

== system ACC_speed_change_curve_cs/Audi_A8_1/ACC_System/TIS2 Bend Road/TIS1 HWT Computing/If Action Subsystem ==
  Distance [m] : Inport
  Velocity [m/s] : Inport  Port=2
  Action Port : ActionPort  PropagateVarSize=During execution  ActionType=then
  Product : Product  Inputs=*/  RndMeth=Zero
  HWT [s] : Outport
  wires:
  Distance [m]/1 -> Product/1
  Velocity [m/s]/1 -> Product/2
  Product/1 -> HWT [s]/1

== system ACC_speed_change_curve_cs/Audi_A8_1/ACC_System/TIS2 Bend Road/TIS1 HWT Computing/If Action Subsystem1 ==
  Action Port : ActionPort  PropagateVarSize=During execution  ActionType=else
  Constant : Constant  Value=inf
  Out1 : Outport  InitialOutput=0
  wires:
  Constant/1 -> Out1/1

== system ACC_speed_change_curve_cs/Audi_A8_1/ACC_System/TIS2 Straight Road/Hold/If Action Subsystem ==
  In1 : Inport
  Action Port : ActionPort  InitializeStates=reset  PropagateVarSize=During execution  ActionType=then
  Constant : Constant
  Constant1 : Constant  Value=0
  Discrete-Time Integrator : DiscreteIntegrator  gainval=100  InitialConditionSource=external  InitialConditionSetting=State (most efficient)  SampleTime=Tsensor  LimitOutput=on  UpperSaturationLimit=1  LowerSaturationLimit=0  ICPrevOutput=DiscIntNeverNeededParam  ICPrevScaledInput=DiscIntNeverNeededParam
  Gain3 : Gain  Gain=1e6  OutDataTypeStr=double
  Switch : Switch  Criteria=u2 > Threshold
  Out1 : Outport
  wires:
  Gain3/1 -> Discrete-Time Integrator/1
  In1/1 -> Gain3/1, Switch/2
  Discrete-Time Integrator/1 -> Out1/1
  Switch/1 -> Discrete-Time Integrator/2
  Constant/1 -> Switch/1
  Constant1/1 -> Switch/3

== system ACC_speed_change_curve_cs/Audi_A8_1/ACC_System/TIS2 Straight Road/Hold/If Action Subsystem1 ==
  In1 : Inport
  Action Port : ActionPort  PropagateVarSize=During execution  ActionType=else
  Out1 : Outport
  wires:
  In1/1 -> Out1/1

== system ACC_speed_change_curve_cs/Audi_A8_1/ACC_System/TIS2 Straight Road/TIS2 HWT Computing/If Action Subsystem ==
  Distance [m] : Inport
  Velocity [m/s] : Inport  Port=2
  Action Port : ActionPort  PropagateVarSize=During execution  ActionType=then
  Product : Product  Inputs=*/  RndMeth=Zero
  HWT [s] : Outport
  wires:
  Distance [m]/1 -> Product/1
  Velocity [m/s]/1 -> Product/2
  Product/1 -> HWT [s]/1

== system ACC_speed_change_curve_cs/Audi_A8_1/ACC_System/TIS2 Straight Road/TIS2 HWT Computing/If Action Subsystem1 ==
  HWT demanded [s] : Inport
  Action Port : ActionPort  PropagateVarSize=During execution  ActionType=else
  Gain : Gain  Gain=2*ones(TISdet(2),1)
  Out1 : Outport
  wires:
  Gain/1 -> Out1/1
  HWT demanded [s]/1 -> Gain/1

== system ACC_speed_change_curve_cs/Audi_A8_1/ACC_System/TIS2 Straight Road/TIS2 HWT Computing2/If Action Subsystem ==
  Distance [m] : Inport
  Velocity [m/s] : Inport  Port=2
  Action Port : ActionPort  PropagateVarSize=During execution  ActionType=then
  Product : Product  Inputs=*/  RndMeth=Zero
  HWT [s] : Outport
  wires:
  Distance [m]/1 -> Product/1
  Velocity [m/s]/1 -> Product/2
  Product/1 -> HWT [s]/1

== system ACC_speed_change_curve_cs/Audi_A8_1/ACC_System/TIS2 Straight Road/TIS2 HWT Computing2/If Action Subsystem1 ==
  Action Port : ActionPort  PropagateVarSize=During execution  ActionType=else
  Constant : Constant  Value=inf
  Out1 : Outport  InitialOutput=0
  wires:
  Constant/1 -> Out1/1

== system ACC_speed_change_curve_cs/Audi_A8_1/ACC_System3/TIS1 ACC action/If Action Subsystem/If Action Subsystem ==
  e : Inport
  th_in : Inport  Port=2
  Action Port : ActionPort  PropagateVarSize=During execution  ActionType=then
  Add : Sum  Inputs=+-
  Constant : Constant  Value=0
  Saturation : Saturate  UpperLimit=100  LowerLimit=0
  Subsystem : Subsystem
  Switch : Switch
  brake : Outport  InitialOutput=0
  throttle : Outport  Port=2  InitialOutput=0
  wires:
  Switch/1 -> Saturation/1
  Add/1 -> Switch/2
  th_in/1 -> Add/1, Switch/3
  Constant/1 -> brake/1
  Saturation/1 -> throttle/1
  e/1 -> Subsystem/1(e)
  Subsystem/1(out) -> Add/2, Switch/1

== system ACC_speed_change_curve_cs/Audi_A8_1/ACC_System3/TIS1 ACC action/If Action Subsystem/If Action Subsystem1 ==
  rd : Inport
  e : Inport  Port=2
  Vp : Inport  Port=3
  EGO distance : Inport  Port=4
  HWT_dem : Inport  Port=5
  th_in : Inport  Port=6
  Action Port : ActionPort  PropagateVarSize=During execution  ActionType=else
  Add : Sum  Inputs=+-
  Constant : Constant  Value=drd/3.6
  If : If  SampleTime=Tsensor
  If Action Subsystem : Subsystem  TreatAsAtomicUnit=on
  If Action Subsystem1 : Subsystem  TreatAsAtomicUnit=on
  Merge : Merge
  Merge1 : Merge
  dec : Outport  InitialOutput=0
  throttle : Outport  Port=2  InitialOutput=0
  wires:
  th_in/1 -> If Action Subsystem1/7(th_in)
  Vp/1 -> If Action Subsystem1/5(Vp)
  HWT_dem/1 -> If Action Subsystem1/4(HWT_dem)
  EGO distance/1 -> If Action Subsystem1/3(EGO_distance[m])
  If Action Subsystem1/1(throttle) -> Merge1/2
  If Action Subsystem1/2(brake) -> Merge/2
  Merge1/1 -> throttle/1
  Merge/1 -> dec/1
  If Action Subsystem/2(throttle) -> Merge1/1
  If Action Subsystem/1(deceleration_[m/s2]) -> Merge/1
  e/1 -> If Action Subsystem1/6(e_acc), If Action Subsystem1/2(e [m]), If Action Subsystem/2(e [m])
  If/2 -> If Action Subsystem1/Action
  If/1 -> If Action Subsystem/Action
  Add/1 -> If/1
  Constant/1 -> Add/2
  rd/1 -> If Action Subsystem1/1(rd), If Action Subsystem/1(rd), Add/1

== system ACC_speed_change_curve_cs/Audi_A8_1/ACC_System3/TIS1 ACC action/If Action Subsystem1/If Action Subsystem ==
  Action Port : ActionPort  PropagateVarSize=During execution  ActionType=then
  Constant : Constant  Value=0
  Constant1 : Constant  Value=0
  dec : Outport  InitialOutput=0
  throttle : Outport  Port=2  InitialOutput=0
  wires:
  Constant1/1 -> throttle/1
  Constant/1 -> dec/1

== system ACC_speed_change_curve_cs/Audi_A8_1/ACC_System3/TIS1 ACC action/If Action Subsystem1/If Action Subsystem1 ==
  rd : Inport
  e : Inport  Port=2
  Vp : Inport  Port=3
  Ego distance : Inport  Port=4
  HWT dem : Inport  Port=5
  Action Port : ActionPort  PropagateVarSize=During execution  ActionType=else
  Add : Sum  Inputs=+-
  Constant : Constant  Value=drd/3.6
  If : If  SampleTime=Tsensor
  If Action Subsystem : Subsystem  TreatAsAtomicUnit=on
  If Action Subsystem1 : Subsystem  TreatAsAtomicUnit=on
  Merge : Merge
  Merge1 : Merge
  dec : Outport  InitialOutput=0
  throttle : Outport  Port=2  InitialOutput=0
  wires:
  HWT dem/1 -> If Action Subsystem1/4(HWT_dem)
  Ego distance/1 -> If Action Subsystem1/3(EGO_distance[m])
  If Action Subsystem1/1(throttle) -> Merge1/2
  If Action Subsystem1/2(brake) -> Merge/2
  Merge1/1 -> throttle/1
  Merge/1 -> dec/1
  If Action Subsystem/2(throttle) -> Merge1/1
  If Action Subsystem/1(dec) -> Merge/1
  Vp/1 -> If Action Subsystem1/5(Vp)
  e/1 -> If Action Subsystem1/2(e [m])
  If/2 -> If Action Subsystem1/Action
  If/1 -> If Action Subsystem/Action
  Add/1 -> If/1
  Constant/1 -> Add/2
  rd/1 -> If Action Subsystem1/1(rd), Add/1

== system ACC_speed_change_curve_cs/Audi_A8_1/ACC_System3/TIS1 Bend Road/Hold/If Action Subsystem ==
  In1 : Inport
  Action Port : ActionPort  InitializeStates=reset  PropagateVarSize=During execution  ActionType=then
  Constant : Constant
  Constant1 : Constant  Value=0
  Discrete-Time Integrator : DiscreteIntegrator  gainval=100  InitialConditionSource=external  InitialConditionSetting=State (most efficient)  SampleTime=Tsensor  LimitOutput=on  UpperSaturationLimit=1  LowerSaturationLimit=0  ICPrevOutput=DiscIntNeverNeededParam  ICPrevScaledInput=DiscIntNeverNeededParam
  Gain3 : Gain  Gain=1e6  OutDataTypeStr=double
  Switch : Switch  Criteria=u2 > Threshold
  Out1 : Outport
  wires:
  Constant1/1 -> Switch/3
  Constant/1 -> Switch/1
  Switch/1 -> Discrete-Time Integrator/2
  Discrete-Time Integrator/1 -> Out1/1
  In1/1 -> Switch/2, Gain3/1
  Gain3/1 -> Discrete-Time Integrator/1

== system ACC_speed_change_curve_cs/Audi_A8_1/ACC_System3/TIS1 Bend Road/Hold/If Action Subsystem1 ==
  In1 : Inport
  Action Port : ActionPort  PropagateVarSize=During execution  ActionType=else
  Out1 : Outport
  wires:
  In1/1 -> Out1/1

== system ACC_speed_change_curve_cs/Audi_A8_1/ACC_System3/TIS1 Bend Road/TIS1 HWT Computing/If Action Subsystem ==
  Distance [m] : Inport
  Velocity [m/s] : Inport  Port=2
  Action Port : ActionPort  PropagateVarSize=During execution  ActionType=then
  Product : Product  Inputs=*/  RndMeth=Zero
  HWT [s] : Outport
  wires:
  Product/1 -> HWT [s]/1
  Velocity [m/s]/1 -> Product/2
  Distance [m]/1 -> Product/1

== system ACC_speed_change_curve_cs/Audi_A8_1/ACC_System3/TIS1 Bend Road/TIS1 HWT Computing/If Action Subsystem1 ==
  Action Port : ActionPort  PropagateVarSize=During execution  ActionType=else
  Constant : Constant  Value=inf
  Out1 : Outport  InitialOutput=0
  wires:
  Constant/1 -> Out1/1

== system ACC_speed_change_curve_cs/Audi_A8_1/ACC_System3/TIS1 Straight Road/Hold/If Action Subsystem ==
  In1 : Inport
  Action Port : ActionPort  InitializeStates=reset  PropagateVarSize=During execution  ActionType=then
  Constant : Constant
  Constant1 : Constant  Value=0
  Discrete-Time Integrator : DiscreteIntegrator  gainval=100  InitialConditionSource=external  InitialConditionSetting=State (most efficient)  SampleTime=Tsensor  LimitOutput=on  UpperSaturationLimit=1  LowerSaturationLimit=0  ICPrevOutput=DiscIntNeverNeededParam  ICPrevScaledInput=DiscIntNeverNeededParam
  Gain3 : Gain  Gain=1e6  OutDataTypeStr=double
  Switch : Switch  Criteria=u2 > Threshold
  Out1 : Outport
  wires:
  Constant1/1 -> Switch/3
  Constant/1 -> Switch/1
  Switch/1 -> Discrete-Time Integrator/2
  Discrete-Time Integrator/1 -> Out1/1
  In1/1 -> Switch/2, Gain3/1
  Gain3/1 -> Discrete-Time Integrator/1

== system ACC_speed_change_curve_cs/Audi_A8_1/ACC_System3/TIS1 Straight Road/Hold/If Action Subsystem1 ==
  In1 : Inport
  Action Port : ActionPort  PropagateVarSize=During execution  ActionType=else
  Out1 : Outport
  wires:
  In1/1 -> Out1/1

== system ACC_speed_change_curve_cs/Audi_A8_1/ACC_System3/TIS1 Straight Road/TIS1 HWT Computing/If Action Subsystem ==
  Distance [m] : Inport
  Velocity [m/s] : Inport  Port=2
  Action Port : ActionPort  PropagateVarSize=During execution  ActionType=then
  Product : Product  Inputs=*/  RndMeth=Zero
  HWT [s] : Outport
  wires:
  Product/1 -> HWT [s]/1
  Velocity [m/s]/1 -> Product/2
  Distance [m]/1 -> Product/1

== system ACC_speed_change_curve_cs/Audi_A8_1/ACC_System3/TIS1 Straight Road/TIS1 HWT Computing/If Action Subsystem1 ==
  HWT demanded [s] : Inport
  Action Port : ActionPort  PropagateVarSize=During execution  ActionType=else
  Gain : Gain  Gain=2*ones(TISdet(1),1)
  Out1 : Outport
  wires:
  HWT demanded [s]/1 -> Gain/1
  Gain/1 -> Out1/1

== system ACC_speed_change_curve_cs/Audi_A8_1/ACC_System3/TIS1 Straight Road/TIS1 HWT Computing1/If Action Subsystem ==
  Distance [m] : Inport
  Velocity [m/s] : Inport  Port=2
  Action Port : ActionPort  PropagateVarSize=During execution  ActionType=then
  Product : Product  Inputs=*/  RndMeth=Zero
  HWT [s] : Outport
  wires:
  Product/1 -> HWT [s]/1
  Velocity [m/s]/1 -> Product/2
  Distance [m]/1 -> Product/1

== system ACC_speed_change_curve_cs/Audi_A8_1/ACC_System3/TIS1 Straight Road/TIS1 HWT Computing1/If Action Subsystem1 ==
  Action Port : ActionPort  PropagateVarSize=During execution  ActionType=else
  Constant : Constant  Value=inf
  Out1 : Outport  InitialOutput=0
  wires:
  Constant/1 -> Out1/1

== system ACC_speed_change_curve_cs/Audi_A8_1/ACC_System3/TIS2 ACC action/If Action Subsystem/If Action Subsystem ==
  e : Inport
  th_in : Inport  Port=2
  Action Port : ActionPort  PropagateVarSize=During execution  ActionType=then
  Add : Sum  Inputs=+-
  Constant : Constant  Value=0
  Rate Limiter : RateLimiter  RisingSlewLimit=BrakeRateMax  FallingSlewLimit=-BrakeRateMax  SampleTimeMode=inherited
  Saturation : Saturate  UpperLimit=100  LowerLimit=0
  Subsystem : Subsystem
  Switch : Switch
  brake : Outport  InitialOutput=0
  throttle : Outport  Port=2  InitialOutput=0
  wires:
  Switch/1 -> Saturation/1
  Add/1 -> Switch/2
  th_in/1 -> Switch/3, Add/1
  Rate Limiter/1 -> throttle/1
  Constant/1 -> brake/1
  Saturation/1 -> Rate Limiter/1
  e/1 -> Subsystem/1(e)
  Subsystem/1(out) -> Switch/1, Add/2

== system ACC_speed_change_curve_cs/Audi_A8_1/ACC_System3/TIS2 ACC action/If Action Subsystem/If Action Subsystem1 ==
  rd : Inport
  e : Inport  Port=2
  Vp : Inport  Port=3
  EGO distance : Inport  Port=4
  HWT_dem : Inport  Port=5
  th_in : Inport  Port=6
  Action Port : ActionPort  PropagateVarSize=During execution  ActionType=else
  Add : Sum  Inputs=+-
  Constant : Constant  Value=drd/3.6
  If : If
  If Action Subsystem : Subsystem  TreatAsAtomicUnit=on
  If Action Subsystem1 : Subsystem  TreatAsAtomicUnit=on
  Merge : Merge
  Merge1 : Merge
  dec : Outport  InitialOutput=0
  throttle : Outport  Port=2  InitialOutput=0
  wires:
  th_in/1 -> If Action Subsystem1/7(th_in)
  Vp/1 -> If Action Subsystem1/5(Vp)
  HWT_dem/1 -> If Action Subsystem1/4(HWT_dem)
  EGO distance/1 -> If Action Subsystem1/3(EGO_distance[m])
  If Action Subsystem1/1(throttle) -> Merge1/2
  If Action Subsystem1/2(brake) -> Merge/2
  Merge1/1 -> throttle/1
  Merge/1 -> dec/1
  If Action Subsystem/2(throttle) -> Merge1/1
  If Action Subsystem/1(deceleration_[m/s2]) -> Merge/1
  e/1 -> If Action Subsystem1/6(e_acc), If Action Subsystem1/2(e [m]), If Action Subsystem/2(e [m])
  If/2 -> If Action Subsystem1/Action
  If/1 -> If Action Subsystem/Action
  Add/1 -> If/1
  Constant/1 -> Add/2
  rd/1 -> If Action Subsystem1/1(rd), If Action Subsystem/1(rd), Add/1

== system ACC_speed_change_curve_cs/Audi_A8_1/ACC_System3/TIS2 ACC action/If Action Subsystem1/If Action Subsystem ==
  Action Port : ActionPort  PropagateVarSize=During execution  ActionType=then
  Constant : Constant  Value=0
  Constant1 : Constant  Value=0
  dec : Outport  InitialOutput=0
  throttle : Outport  Port=2  InitialOutput=0
  wires:
  Constant1/1 -> throttle/1
  Constant/1 -> dec/1

== system ACC_speed_change_curve_cs/Audi_A8_1/ACC_System3/TIS2 ACC action/If Action Subsystem1/If Action Subsystem1 ==
  rd : Inport
  e : Inport  Port=2
  Vp : Inport  Port=3
  Ego distance : Inport  Port=4
  HWT dem : Inport  Port=5
  Action Port : ActionPort  PropagateVarSize=During execution  ActionType=else
  Add : Sum  Inputs=+-
  Constant : Constant  Value=drd/3.6
  If : If
  If Action Subsystem : Subsystem  TreatAsAtomicUnit=on
  If Action Subsystem1 : Subsystem  TreatAsAtomicUnit=on
  Merge : Merge
  Merge1 : Merge
  dec : Outport  InitialOutput=0
  throttle : Outport  Port=2  InitialOutput=0
  wires:
  HWT dem/1 -> If Action Subsystem1/4(HWT_dem)
  Ego distance/1 -> If Action Subsystem1/3(EGO_distance[m])
  If Action Subsystem1/1(throttle) -> Merge1/2
  If Action Subsystem1/2(brake) -> Merge/2
  Merge1/1 -> throttle/1
  Merge/1 -> dec/1
  If Action Subsystem/2(throttle) -> Merge1/1
  If Action Subsystem/1(dec) -> Merge/1
  Vp/1 -> If Action Subsystem1/5(Vp)
  e/1 -> If Action Subsystem1/2(e [m])
  If/2 -> If Action Subsystem1/Action
  If/1 -> If Action Subsystem/Action
  Add/1 -> If/1
  Constant/1 -> Add/2
  rd/1 -> If Action Subsystem1/1(rd), Add/1

== system ACC_speed_change_curve_cs/Audi_A8_1/ACC_System3/TIS2 ACC action/Stop & Go/If Action Subsystem ==
  TIS2_Distance[m] : Inport
  TIS2_Safe_Distance [m] : Inport  Port=2
  rd : Inport  Port=3
  th_in : Inport  Port=4
  Vp : Inport  Port=5
  Stand : Inport  Port=6
  Action Port : ActionPort  PropagateVarSize=During execution  ActionType=then
  Add2 : Sum  Inputs=-+
  If : If
  If Action Subsystem : Subsystem  TreatAsAtomicUnit=on
  If Action Subsystem1 : Subsystem  TreatAsAtomicUnit=on
  Merge : Merge
  Merge1 : Merge
  Stand1 : InportShadow  Port=6
  br : Outport
  th : Outport  Port=2
  wires:
  th_in/1 -> If Action Subsystem/3(th_in)
  Stand1/1 -> If Action Subsystem1/5(stand)
  Stand/1 -> If Action Subsystem/5(Stand)
  Vp/1 -> If Action Subsystem1/3(Vp)
  If Action Subsystem1/2(throttle1) -> Merge1/1
  If Action Subsystem1/1(brake) -> Merge/2
  If Action Subsystem/2(throttle) -> Merge1/2
  If Action Subsystem/1(brake) -> Merge/1
  Merge/1 -> br/1
  Merge1/1 -> th/1
  rd/1 -> If Action Subsystem1/1(rd1), If Action Subsystem/1(rd)
  If/1 -> If Action Subsystem/Action
  If/2 -> If Action Subsystem1/Action
  Add2/1 -> If Action Subsystem1/2(e [m]), If Action Subsystem/2(e [m]), If/1
  TIS2_Safe_Distance [m]/1 -> Add2/1
  TIS2_Distance[m]/1 -> If Action Subsystem1/4(dis), If Action Subsystem/4(dis), Add2/2

== system ACC_speed_change_curve_cs/Audi_A8_1/ACC_System3/TIS2 ACC action/Stop & Go/If Action Subsystem1 ==
  In1 : Inport
  In2 : Inport  Port=2
  Action Port : ActionPort  PropagateVarSize=During execution  ActionType=else
  Out1 : Outport
  Out2 : Outport  Port=2
  wires:
  In2/1 -> Out2/1
  In1/1 -> Out1/1
